simulink model "simplifiedtester"  (R2014b)
settings: Solver=ode45  StartTime=0.0  StopTime=10.0  RelTol=1e-3
values from neighbouring files (symbols this model uses):
  a0 = ((Rt1*cs1*cs2+cs1*(Rt2*cs2+cs1*(Rt2*cs2+Rt3*cs2))))/(cs1*cs2)    (= 5000100)    [przypadkowy_kod.m]
  a1 = ((I1*cs1*cs2+Rt1*(Rt3*cs1+Rt2*cs2+Rt3*cs2)+cs1*(Rt1+Rt2+I3*cs2+I3*cs2+I2*cs2+I3*cs1)))/(cs1*cs2)    (= 5.152)    [przypadkowy_kod.m]    (also in zmiennefuruta.m = 0)
  a2 = (I1*(Rt3*cs1+Rt2*cs2+Rt3*cs2)+Rt1*(Rt2*Rt3+I3*cs2+I2*cs2+I3*cs1)+cs1*(I2*Rt3+I3*Rt2))/(cs1*cs2)    (= 0.00805)    [przypadkowy_kod.m]    (also in zmiennefuruta.m = -44.5909090909)
  a3 = ((I1*(Rt2*Rt3+I3*cs2+I2*cs2+I3*cs1)+Rt1*(I2*Rt3+I3*Rt2)+cs1*I2*I3))/(cs1*cs2)    (= 8.3e-05)    [przypadkowy_kod.m]    (also in zmiennefuruta.m = 4.41818181818)
  a4 = ((I1*(I1*Rt3+I3*Rt2)+Rt1*I2*I3))/(cs1*cs2)    (= 6e-08)    [przypadkowy_kod.m]    (also in zmiennefuruta.m = 8.57857738592)
  a5 = (I1*I2*I3)/(cs1*cs2)    (= 4e-10)    [przypadkowy_kod.m]    (also in zmiennefuruta.m = 5.95734540689)
settings Model: Creator=Jacek  LastModifiedBy=tehKa

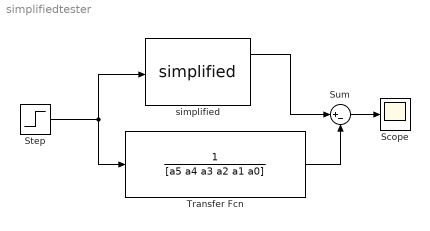
== system simplifiedtester ==
  Scope : Scope
  Step : Step  Time=0  After=100  SampleTime=0
  Sum : Sum  Inputs=|+-
  Transfer Fcn : TransferFcn  Denominator=[a5 a4 a3 a2 a1 a0]
  simplified : S-Function  FunctionName=simplified  EnableBusSupport=off
      mask Display: port_label('input',1,'Torque.'); port_label('output',1,'omega3.'); port_label('output',2,'DEBUG')
  wires:
  Sum/1 -> Scope/1
  Transfer Fcn/1 -> Sum/2
  simplified/1 -> Sum/1
  Step/1 -> Transfer Fcn/1, simplified/1
